simulink model "D53_LKAS_JLU_20200910_1510"  (R2018b)
settings: Solver=ode3  StartTime=0.0  StopTime=10.0  FixedStep=0.01  RelTol=1e-3  EnableMultiTasking=on
model workspace (MAT data in the model file):
  MCOS : class17 (value not decoded)
  MCOS : class17 (value not decoded)
  MCOS : class17 (value not decoded)
  MCOS : class17 (value not decoded)
  MCOS : class17 (value not decoded)
  MCOS : class17 (value not decoded)
  MCOS : class17 (value not decoded)
  MCOS : class17 (value not decoded)
  MCOS : class17 (value not decoded)
  MCOS : class17 (value not decoded)
  MCOS : class17 (value not decoded)
  MCOS : class17 (value not decoded)
  MCOS : class17 (value not decoded)
  MCOS : class17 (value not decoded)
  MCOS : class17 (value not decoded)
  MCOS : class17 (value not decoded)
  MCOS : class17 (value not decoded)
  MCOS : class17 (value not decoded)
  MCOS : class17 (value not decoded)
  MCOS : class17 (value not decoded)
  MCOS : class17 (value not decoded)
  MCOS : class17 (value not decoded)
  MCOS : class17 (value not decoded)
  MCOS : class17 (value not decoded)
  MCOS : class17 (value not decoded)
  MCOS : class17 (value not decoded)
  MCOS : class17 (value not decoded)
  MCOS : class17 (value not decoded)
  MCOS : class17 (value not decoded)
  MCOS : class17 (value not decoded)
  MCOS : class17 (value not decoded)
  MCOS : class17 (value not decoded)
  MCOS : class17 (value not decoded)
  MCOS : class17 (value not decoded)
  MCOS : class17 (value not decoded)
  MCOS : class17 (value not decoded)
  MCOS : class17 (value not decoded)
  MCOS : class17 (value not decoded)
  MCOS : class17 (value not decoded)
  MCOS : class17 (value not decoded)
  MCOS : class17 (value not decoded)
  MCOS : class17 (value not decoded)
  MCOS : class17 (value not decoded)
  MCOS : class17 (value not decoded)
  MCOS : class17 (value not decoded)
  MCOS : class17 (value not decoded)
  MCOS : class17 (value not decoded)
  MCOS : class17 (value not decoded)
  MCOS : class17 (value not decoded)
  MCOS : class17 (value not decoded)
  MCOS : class17 (value not decoded)
  MCOS : class17 (value not decoded)
  MCOS : class17 (value not decoded)
  MCOS : class17 (value not decoded)
  MCOS : class17 (value not decoded)
  MCOS : class17 (value not decoded)
  MCOS : class17 (value not decoded)
  MCOS : class17 (value not decoded)
  MCOS : class17 (value not decoded)
  MCOS : class17 (value not decoded)
  MCOS : class17 (value not decoded)
  MCOS : class17 (value not decoded)
  MCOS : class17 (value not decoded)
  MCOS : class17 (value not decoded)
  MCOS : class17 (value not decoded)
  MCOS : class17 (value not decoded)
  MCOS : class17 (value not decoded)
  MCOS : class17 (value not decoded)
  MCOS : class17 (value not decoded)
  MCOS : class17 (value not decoded)
  MCOS : class17 (value not decoded)
  MCOS : class17 (value not decoded)
  MCOS : class17 (value not decoded)
  MCOS : class17 (value not decoded)
  MCOS : class17 (value not decoded)
  MCOS : class17 (value not decoded)
  MCOS : class17 (value not decoded)
  MCOS : class17 (value not decoded)
  MCOS : class17 (value not decoded)
  MCOS : class17 (value not decoded)
  MCOS : class17 (value not decoded)
  MCOS : class17 (value not decoded)
  MCOS : class17 (value not decoded)
  MCOS : class17 (value not decoded)
  MCOS : class17 (value not decoded)
  MCOS : class17 (value not decoded)
  MCOS : class17 (value not decoded)
  MCOS : class17 (value not decoded)
  MCOS : class17 (value not decoded)
undefined symbols (not defined in the file): LKA_CarWidth, LKA_SampleTime, LKA_StrRatio_C, LKA_Veh2CamL_C, LKA_Veh2CamW_C, LKA_WhlBaseL_C, LL_CompSWA_C, LL_CrvtPrvwT_C, LL_DesDvt_C, LL_DvtComp_C, LL_DvtPrvwT_C, LL_DvtSpdDet_vDvtSpdMin_C, LL_HdAgExT_C, LL_HdAgPrvwT_C, LL_LAccMax_C, LL_LAccRMax_C, LL_LDW_EarliestWarnLine_C, LL_LDW_LatestWarnLine_C, LL_LDWS_SUPPRESS_HEADING, LL_LFClb_TFC_DiffCtlBalance, LL_LFClb_TFC_DiffCtrlMaxSWA, LL_LFClb_TFC_DiffCtrlRatio, LL_LFClb_TFC_facmGainLutGain1_C, LL_LFClb_TFC_facmGainLutGain2_C, LL_LFClb_TFC_facmIntegRatio, LL_LFClb_TFC_facmKlat_C, LL_LFClb_TFC_FfCtlRatio_C, LL_LFClb_TFC_phiIntegCtlMaxSWA_C, LL_LFClb_TFC_tiKlatPrvwT_C, LL_LFClb_TFC_vGainLutVehSpdLwr_C, LL_LFClb_TFC_vGainLutVehSpdUpr_C, LL_LKA_EarliestWarnLine_C, LL_LKA_LatestWarnLine_C, LL_LKAExPrcs_ExitC0Dvt, LL_LKAExPrcs_ExitC0Swt, LL_LKAExPrcs_tiExitTime1, LL_LKAExPrcs_tiExitTime2, LL_LKAExPrcs_tiExitTime3, LL_LKAS_OUT_OF_CONTROL_LAT_VEL, LL_LKAS_OUT_OF_CONTROL_TTLC, LL_LKASWASyn_M0, LL_LKASWASyn_M1, LL_LKASWASyn_M2, LL_LKASWASyn_M3K, LL_LKASWASyn_SWAaddMax, LL_LKASWASyn_T2, LL_LKASWASyn_tiTrqSwaRtTime, LL_LKASWASyn_tiTrqSwaTime, LL_LKASWASyn_TrqMax, LL_LKASWASyn_TrqSwaAddSwt, LL_LKASWASyn_TrqSwaRateDiff, LL_LSpdCompT_C, LL_lStpLngth_C, LL_MAX_DELAY_EPSSTAR_TIME, LL_MAX_DRIVER_TORQUE_DISABLE, LL_MAX_DRIVER_TORQUE_ENABLE, LL_MAX_LANE_WIDTH_DISABLE, LL_MAX_LANE_WIDTH_ENABLE, LL_MAX_LAT_ACC_DISABLE, LL_MAX_LAT_ACC_ENABLE ... (+30)
libraries: simulink x134, canmsglib x52, dspstat3 x3, simulink_extras x1
(part 9 of 18)

== system D53_LKAS_JLU_20200910_1510/LL/LLOn/LKA Input Processing (LKAInP)/Predicted Heading Angle Calculation (PrHdAg) ==
  PrHdAg_bsTTLCInfo : Inport
  PrdcHdAg_stLKAActvFlg : Inport  Port=2
  PrHdAg_bsInInfoSyn : Inport  Port=3
  PrHdAg_bsLKAClb : Inport  Port=4
  Add : Sum  OutDataTypeStr=single
  Add1 : Sum  OutDataTypeStr=single
  Bus Creator : BusCreator  Inputs=10
  Bus Selector : BusSelector  OutputSignals=bsLaneInfo.bsL0Info,bsVehMovInfo.ESC_VehSpd,bsLaneInfo.bsR0Info,bsSWAInfo.SW_Angle
  Bus Selector1 : BusSelector  OutputSignals=LL_HdAgPrvwT_C
  Bus Selector2 : BusSelector  OutputSignals=LFTTTLC,RGTTTLC
  Heading Angle (HdAg) : Subsystem
  Lane Information Selection (LaneInfoSel) : Subsystem
  Lane Information Selection (LaneInfoSel)1 : Subsystem
  Min : MinMax  Inputs=2
  Perdicted Heading Angle Compensation (PrdcHdAgComp) : Subsystem
  Perdicted Heading Angle from Right Lane Line (PrdcHdAgRgt) : Subsystem
  Perdicted Heading Angle from Right Lane Line (PrdcHdAgRgt)1 : Subsystem
  Predicted Heading Angle from Left Lane Line (PrdcHdAgtLft) : Subsystem
  Predicted Heading Angle from Left Lane Line (PrdcHdAgtLft)1 : Subsystem
  Saturation : Saturate  UpperLimit=2  LowerLimit=0.5
  Z Calculation (ZCalc) : Subsystem
  Z Calculation (ZCalc)1 : Subsystem
  PrHdAg_bsPrHdAgInfo : Outport
  wires:
  Perdicted Heading Angle from Right Lane Line (PrdcHdAgRgt)1/1(PrdcHdAgRgt_phiPrdcHdAgRgt) -> Bus Creator/10  "phiPrvwHdAgRgt"
  Predicted Heading Angle from Left Lane Line (PrdcHdAgtLft)1/1(PrdcHdAgtLft_phiPrdcHdAgLft) -> Bus Creator/9  "phiPrvwHdAgLft"
  Z Calculation (ZCalc)1/1(ZCalc_lPrvwDstZ) -> Predicted Heading Angle from Left Lane Line (PrdcHdAgtLft)1/2(PrdcHdAgtLft_lPrvwDstZ), Perdicted Heading Angle from Right Lane Line (PrdcHdAgRgt)1/1(PrdcHdAgRgt_lPrvwDstZ)
  Bus Selector1/1 -> Z Calculation (ZCalc)1/2(ZCalc_tiHdAgPrvwT_C)  "<LL_HdAgPrvwT_C>"
  PrHdAg_bsLKAClb/1 -> Bus Selector1/1
  Heading Angle (HdAg)/3(HdAg_phiHdAgRgt) -> Bus Creator/8  "phiHdAgRgt"
  Heading Angle (HdAg)/2(HdAg_phiHdAgLft) -> Bus Creator/7  "phiHdAgLft"
  Heading Angle (HdAg)/1(HdAg_phiHdAg) -> Bus Creator/6  "phiHdAg"
  Saturation/1 -> Perdicted Heading Angle Compensation (PrdcHdAgComp)/3(PrdcHdAgComp_tiHdAgPrvwT_C), Z Calculation (ZCalc)/2(ZCalc_tiHdAgPrvwT_C)
  Bus Selector2/2 -> Min/2  "<RGTTTLC>"
  Bus Selector2/1 -> Min/1  "<LFTTTLC>"
  PrHdAg_bsTTLCInfo/1 -> Bus Selector2/1
  Lane Information Selection (LaneInfoSel)1/1(LaneInfoSel_facmActvLane) -> Bus Creator/2  "phiPrvwTTLCHdAg"
  Bus Selector/1 -> Predicted Heading Angle from Left Lane Line (PrdcHdAgtLft)/1(PrdcHdAgtLft_bsL0Info), Predicted Heading Angle from Left Lane Line (PrdcHdAgtLft)1/1(PrdcHdAgtLft_bsL0Info)  "<bsL0Info>"
  Z Calculation (ZCalc)/1(ZCalc_lPrvwDstZ) -> Predicted Heading Angle from Left Lane Line (PrdcHdAgtLft)/2(PrdcHdAgtLft_lPrvwDstZ), Perdicted Heading Angle from Right Lane Line (PrdcHdAgRgt)/1(PrdcHdAgRgt_lPrvwDstZ)
  Lane Information Selection (LaneInfoSel)/1(LaneInfoSel_facmActvLane) -> Bus Creator/1  "phiPrdcTTLCHdAg"
  PrdcHdAg_stLKAActvFlg/1 -> Lane Information Selection (LaneInfoSel)/1(LaneInfoSel_stLKAActvFlg), Lane Information Selection (LaneInfoSel)1/1(LaneInfoSel_stLKAActvFlg)
  Add1/1 -> Lane Information Selection (LaneInfoSel)/3(LaneInfoSel_facmRgtLane)  "phiPrdcHdAgRgt"
  Add/1 -> Lane Information Selection (LaneInfoSel)/2(LaneInfoSel_facmLftLane)  "phiPrdcHdAgLft"
  Perdicted Heading Angle Compensation (PrdcHdAgComp)/1(PrdcHdAgComp_phiPrdcHdAgComp) -> Add1/2, Bus Creator/5, Add/2  "phiPrdcHdAgComp"
  Predicted Heading Angle from Left Lane Line (PrdcHdAgtLft)/1(PrdcHdAgtLft_phiPrdcHdAgLft) -> Add/1, Bus Creator/3, Lane Information Selection (LaneInfoSel)1/2(LaneInfoSel_facmLftLane)  "phiPrvwTTLCHdAgLft"
  Perdicted Heading Angle from Right Lane Line (PrdcHdAgRgt)/1(PrdcHdAgRgt_phiPrdcHdAgRgt) -> Add1/1, Lane Information Selection (LaneInfoSel)1/3(LaneInfoSel_facmRgtLane), Bus Creator/4  "phiPrvwTTLCHdAgRgt"
  Bus Creator/1 -> PrHdAg_bsPrHdAgInfo/1
  PrHdAg_bsInInfoSyn/1 -> Bus Selector/1, Heading Angle (HdAg)/1(HdAg_bsLaneInfo)
  Bus Selector/2 -> Z Calculation (ZCalc)/1(ZCalc_vVehSpd), Perdicted Heading Angle Compensation (PrdcHdAgComp)/1(PrdcHdAgComp_vVehSpd), Z Calculation (ZCalc)1/1(ZCalc_vVehSpd)  "<ESC_VehSpd>"
  Bus Selector/3 -> Perdicted Heading Angle from Right Lane Line (PrdcHdAgRgt)/2(PrdcHdAgRgt_bsR0Info), Perdicted Heading Angle from Right Lane Line (PrdcHdAgRgt)1/2(PrdcHdAgRgt_bsR0Info)  "<bsR0Info>"
  Bus Selector/4 -> Perdicted Heading Angle Compensation (PrdcHdAgComp)/2(PrdcHdAgComp_phiSWA)  "<SW_Angle>"
  Min/1 -> Saturation/1

== system D53_LKAS_JLU_20200910_1510/LL/LLOn/LKA Input Processing (LKAInP)/Previewed Curvature (PrCrvt) ==
  PrvwCrvt_stLKAActvFlg : Inport
  PrvwCrvt_bsInInfoSyn : Inport  Port=2
  PrvwCrvt_tiCrvtPrvwT_C : Inport  Port=3
  Bus Creator : BusCreator  Inputs=3
  Bus Selector : BusSelector  OutputSignals=LL_CrvtPrvwT_C
  Bus Selector2 : BusSelector  OutputSignals=bsLaneInfo.bsL0Info,bsVehMovInfo.ESC_VehSpd,bsLaneInfo.bsR0Info
  Curvature Ahead of Left Lane Line (CrvtAhdLft) : Subsystem
  Curvature Ahead of Left Lane Line (CrvtAhdLft)1 : Subsystem
  Lane Information Selection (LaneInfoSel) : Subsystem
  Z Calculation (ZCalc) : Subsystem
  PrvwCrvt_bsPrvwCrvtInfo : Outport
  wires:
  Bus Creator/1 -> PrvwCrvt_bsPrvwCrvtInfo/1
  Lane Information Selection (LaneInfoSel)/1(LaneInfoSel_facmActvLane) -> Bus Creator/1  "crPrvwCrvt"
  Curvature Ahead of Left Lane Line (CrvtAhdLft)1/1(CrvtAhdRgt_crCrvtAhdRgt) -> Bus Creator/3, Lane Information Selection (LaneInfoSel)/3(LaneInfoSel_facmRgtLane)  "crPrvwCrvtRgt"
  Curvature Ahead of Left Lane Line (CrvtAhdLft)/1(CrvtAhdLft_crCrvtAhdLft) -> Lane Information Selection (LaneInfoSel)/2(LaneInfoSel_facmLftLane), Bus Creator/2  "crPrvwCrvtLft"
  PrvwCrvt_stLKAActvFlg/1 -> Lane Information Selection (LaneInfoSel)/1(LaneInfoSel_stLKAActvFlg)
  Bus Selector/1 -> Z Calculation (ZCalc)/2(ZCalc_tiCrvtPrvwT_C)  "<LL_CrvtPrvwT_C>"
  PrvwCrvt_tiCrvtPrvwT_C/1 -> Bus Selector/1
  Bus Selector2/2 -> Z Calculation (ZCalc)/1(ZCalc_vVehSpd)  "<ESC_VehSpd>"
  Bus Selector2/3 -> Curvature Ahead of Left Lane Line (CrvtAhdLft)1/2(CrvtAhdRgt_bsR0Info)  "<bsR0Info>"
  Bus Selector2/1 -> Curvature Ahead of Left Lane Line (CrvtAhdLft)/1(CrvtAhdLft_bsL0Info)  "<bsL0Info>"
  Z Calculation (ZCalc)/1(ZCalc_lPrvwDstZ) -> Curvature Ahead of Left Lane Line (CrvtAhdLft)/2(CrvtAhdLft_lPrvwDstZ), Curvature Ahead of Left Lane Line (CrvtAhdLft)1/1(CrvtAhdRgt_lPrvwDstZ)
  PrvwCrvt_bsInInfoSyn/1 -> Bus Selector2/1

== system D53_LKAS_JLU_20200910_1510/LL/LLOn/LKA Input Processing (LKAInP)/Steering Wheel Position Calculation (SWAPosCal) ==
  SWAPosCal_bsInInfoSyn : Inport
  Bus Selector : BusSelector  OutputSignals=bsLaneInfo.bsL0Info,bsLaneInfo.bsR0Info,bsVehMovInfo.ESC_VehSpd,bsSWAInfo.SW_Angle
  Bus Selector2 : BusSelector  OutputSignals=LKA_SampleTime
  Subsystem : Subsystem
  Subsystem1 : Subsystem
  SWAPosCal : Outport
  wires:
  Bus Selector2/1 -> Subsystem/2(<LKA_SampleTime>)  "<LKA_SampleTime>"
  [LLClb_bsConstantClb] -> Bus Selector2/1
  Subsystem/1(SWAPos) -> SWAPosCal/1
  Bus Selector/4 -> Subsystem1/4(SWA), Subsystem/1(SWAIn)  "<SW_Angle>"
  Bus Selector/3 -> Subsystem1/3(VehSpd)  "<ESC_VehSpd>"
  Subsystem1/1(Flg) -> Subsystem/Enable  "SWAPosEna"
  Bus Selector/2 -> Subsystem1/2(R0)  "<bsR0Info>"
  Bus Selector/1 -> Subsystem1/1(L0)  "<bsL0Info>"
  SWAPosCal_bsInInfoSyn/1 -> Bus Selector/1

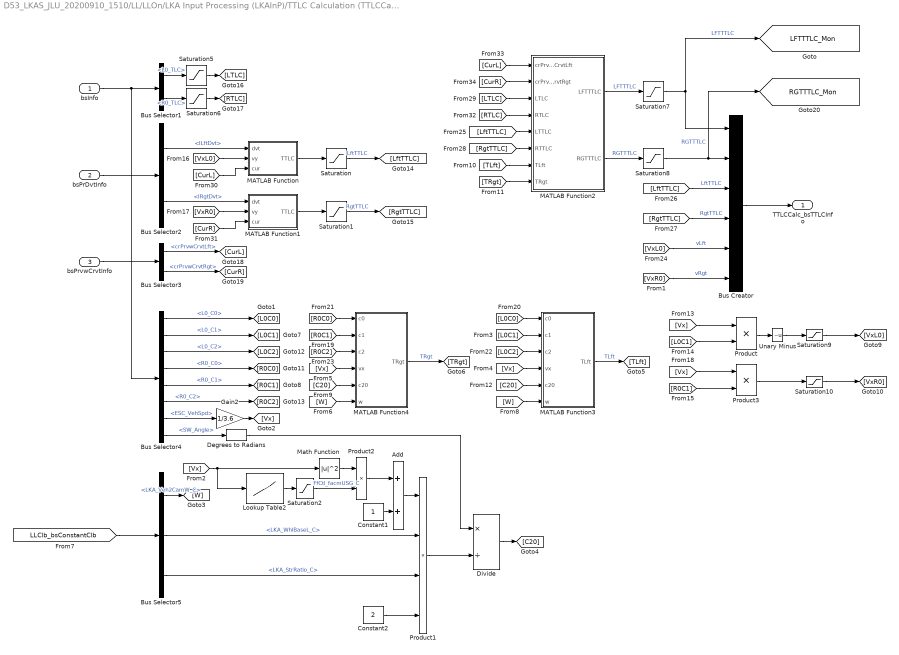
== system D53_LKAS_JLU_20200910_1510/LL/LLOn/LKA Input Processing (LKAInP)/TTLC Calculation (TTLCCalc) ==
  bsInfo : Inport
  bsPrDvtInfo : Inport  Port=2
  bsPrvwCrvtInfo : Inport  Port=3
  Add : Sum  OutDataTypeStr=single
  Bus Creator : BusCreator  Inputs=6
  Bus Selector1 : BusSelector  OutputSignals=bsLaneInfo.bsL0Info.L0_TLC,bsLaneInfo.bsR0Info.R0_TLC
  Bus Selector2 : BusSelector  OutputSignals=ILftDvt,IRgtDvt
  Bus Selector3 : BusSelector  OutputSignals=crPrvwCrvtLft,crPrvwCrvtRgt
  Bus Selector4 : BusSelector  OutputSignals=bsLaneInfo.bsL0Info.L0_C0,bsLaneInfo.bsL0Info.L0_C1,bsLaneInfo.bsL0Info.L0_C2,bsLaneInfo.bsR0Info.R0_C0,bsLaneInfo.bsR0Info.R0_C1,bsLaneInfo.bsR0Info.R0_C2,bsVehMovInfo.ESC_VehSpd,bsSWAInfo.SW_Angle
  Bus Selector5 : BusSelector  OutputSignals=LKA_Veh2CamW_C,LKA_WhlBaseL_C,LKA_StrRatio_C
  Constant1 : Constant  OutDataTypeStr=single
  Constant2 : Constant  Value=2  OutDataTypeStr=single
  Degrees to Radians : simulink_extras/Transformations/Degrees to Radians
  Divide : Product  Inputs=*/
  Gain2 : Gain  Gain=1/3.6
  Lookup Table2 : Lookup_n-D  NumberOfTableDimensions=1  BreakpointsForDimension1=[11.7,18.83,26.98,31.98,51.04,79,86.08,90.59]  BeginIndexSearchUsingPreviousIndexResult=on  Table=[0.012141,0.005179,0.00298,0.002547,0.001715,0.001283,0.001021,0.000982]  DiagnosticForOutOfRangeInput=Warning  RemoveProtectionInput=on  InternalRulePriority=Speed  OutDataTypeStr=single  RndMeth=Simplest  InputSameDT=on
  MATLAB Function : MATLAB Function  TreatAsAtomicUnit=on
  MATLAB Function1 : MATLAB Function  TreatAsAtomicUnit=on
  MATLAB Function2 : MATLAB Function  TreatAsAtomicUnit=on
  MATLAB Function3 : MATLAB Function  TreatAsAtomicUnit=on
  MATLAB Function4 : MATLAB Function  TreatAsAtomicUnit=on
  Math Function : Math  Operator=magnitude^2  OutDataTypeStr=single  SaturateOnIntegerOverflow=on
  Product : Product
  Product1 : Product  Inputs=4  OutDataTypeStr=single
  Product2 : Product  OutDataTypeStr=single
  Product3 : Product
  Saturation : Saturate  UpperLimit=2  LowerLimit=0.6  OutDataTypeStr=single
  Saturation1 : Saturate  UpperLimit=2  LowerLimit=0.6  OutDataTypeStr=single
  Saturation10 : Saturate  UpperLimit=1  LowerLimit=-1
  Saturation2 : Saturate  UpperLimit=0.01  LowerLimit=0
  Saturation5 : Saturate  UpperLimit=2  LowerLimit=0.6
  Saturation6 : Saturate  UpperLimit=2  LowerLimit=0.6
  Saturation7 : Saturate  UpperLimit=2  LowerLimit=0.8
  Saturation8 : Saturate  UpperLimit=2  LowerLimit=0.8
  Saturation9 : Saturate  UpperLimit=1  LowerLimit=-1
  Unary Minus : UnaryMinus
  TTLCCalc_bsTTLCInfo : Outport
  tag scope: LFTTTLC_Mon=global, RGTTTLC_Mon=global
  wires:
  Constant2/1 -> Product1/4
  [CurR] -> MATLAB Function2/2(crPrvwCrvtRgt)
  Saturation8/1 -> Bus Creator/2, [RGTTTLC_Mon]  "RGTTTLC"
  MATLAB Function2/2(RGTTTLC) -> Saturation8/1  "RGTTTLC"
  [LTLC] -> MATLAB Function2/3(LTLC)
  [RgtTTLC] -> MATLAB Function2/6(RTTLC)
  [RgtTTLC] -> Bus Creator/4  "RgtTTLC"
  [RTLC] -> MATLAB Function2/4(RTLC)
  MATLAB Function2/1(LFTTTLC) -> Saturation7/1  "LFTTTLC"
  [CurL] -> MATLAB Function2/1(crPrvwCrvtLft)
  Saturation7/1 -> Bus Creator/1, [LFTTTLC_Mon]  "LFTTTLC"
  [LftTTLC] -> Bus Creator/3  "LftTTLC"
  [TRgt] -> MATLAB Function2/8(TRgt)
  [LftTTLC] -> MATLAB Function2/5(LTTLC)
  [TLft] -> MATLAB Function2/7(TLft)
  Bus Creator/1 -> TTLCCalc_bsTTLCInfo/1
  [VxL0] -> Bus Creator/5  "vLft"
  [VxR0] -> Bus Creator/6  "vRgt"
  Saturation10/1 -> [VxR0]
  Unary Minus/1 -> Saturation9/1
  [R0C1] -> Product3/2
  Product/1 -> Unary Minus/1
  Saturation9/1 -> [VxL0]
  [Vx] -> Product/1
  [L0C1] -> Product/2
  [Vx] -> Product3/1
  Product3/1 -> Saturation10/1
  [L0C0] -> MATLAB Function3/1(c0)
  [L0C2] -> MATLAB Function3/3(c2)
  [Vx] -> MATLAB Function4/4(vx)
  [R0C1] -> MATLAB Function4/2(c1)
  [W] -> MATLAB Function3/6(w)
  [L0C1] -> MATLAB Function3/2(c1)
  MATLAB Function3/1(TLft) -> [TLft]  "TLft"
  [R0C0] -> MATLAB Function4/1(c0)
  [W] -> MATLAB Function4/6(w)
  [C20] -> MATLAB Function4/5(c20)
  [Vx] -> MATLAB Function3/4(vx)
  [R0C2] -> MATLAB Function4/3(c2)
  MATLAB Function4/1(TRgt) -> [TRgt]  "TRgt"
  [C20] -> MATLAB Function3/5(c20)
  Bus Selector4/3 -> [L0C2]  "<L0_C2>"
  Bus Selector4/1 -> [L0C0]  "<L0_C0>"
  Bus Selector4/2 -> [L0C1]  "<L0_C1>"
  Bus Selector4/6 -> [R0C2]  "<R0_C2>"
  Bus Selector4/4 -> [R0C0]  "<R0_C0>"
  Bus Selector4/5 -> [R0C1]  "<R0_C1>"
  Bus Selector3/2 -> [CurR]  "<crPrvwCrvtRgt>"
  Bus Selector3/1 -> [CurL]  "<crPrvwCrvtLft>"
  [CurL] -> MATLAB Function/3(cur)
  [CurR] -> MATLAB Function1/3(cur)
  Bus Selector2/1 -> MATLAB Function/1(dvt)  "<ILftDvt>"
  Saturation1/1 -> [RgtTTLC]  "RgtTTLC"
  Saturation/1 -> [LftTTLC]  "LftTTLC"
  MATLAB Function/1(TTLC) -> Saturation/1
  MATLAB Function1/1(TTLC) -> Saturation1/1
  [VxR0] -> MATLAB Function1/2(vy)
  [VxL0] -> MATLAB Function/2(vy)
  Bus Selector2/2 -> MATLAB Function1/1(dvt)  "<IRgtDvt>"
  Bus Selector1/2 -> Saturation6/1  "<R0_TLC>"
  Bus Selector1/1 -> Saturation5/1  "<L0_TLC>"
  Saturation5/1 -> [LTLC]
  Saturation6/1 -> [RTLC]
  bsPrvwCrvtInfo/1 -> Bus Selector3/1
  bsPrDvtInfo/1 -> Bus Selector2/1
  bsInfo/1 -> Bus Selector4/1, Bus Selector1/1
  [LLClb_bsConstantClb] -> Bus Selector5/1
  Product2/1 -> Add/1
  Math Function/1 -> Product2/1
  Lookup Table2/1 -> Saturation2/1
  Constant1/1 -> Add/2
  Saturation2/1 -> Product2/2  "FfCtl_facmUSG_C"
  Bus Selector4/7 -> Gain2/1  "<ESC_VehSpd>"
  Add/1 -> Product1/1
  Bus Selector5/2 -> Product1/2  "<LKA_WhlBaseL_C>"
  Bus Selector5/3 -> Product1/3  "<LKA_StrRatio_C>"
  Product1/1 -> Divide/2
  Bus Selector4/8 -> Degrees to Radians/1  "<SW_Angle>"
  Degrees to Radians/1 -> Divide/1
  Gain2/1 -> [Vx]
  [Vx] -> Lookup Table2/1, Math Function/1
  Bus Selector5/1 -> [W]  "<LKA_Veh2CamW_C>"
  Divide/1 -> [C20]

== system D53_LKAS_JLU_20200910_1510/LL/LLOn/LKA Input Processing (LKAInP)/Under The Limit (UndrLim) ==
  UndrLim_bsInInfoSyn : Inport
  UndrLim_bsUndrLimClb : Inport  Port=2
  Bus Selector : BusSelector  OutputSignals=LL_LAccMax_C,LL_LAccRMax_C
  Bus Selector1 : BusSelector  OutputSignals=bsVehMovInfo.ESC_VehSpd
  Bus Selector2 : BusSelector  OutputSignals=LKA_StrRatio_C,LKA_WhlBaseL_C
  Saturation : Saturate  UpperLimit=150  LowerLimit=0.001
  Steering Wheel Angel Max (SWAMax) : Subsystem
  Steering Wheel Angel Rate Max (SWARMax) : Subsystem
  UndrLim_phiSWAMax : Outport
  UndrLim_dphiSWARMax : Outport  Port=2
  wires:
  [LLClb_bsConstantClb] -> Bus Selector2/1
  Bus Selector2/2 -> Steering Wheel Angel Rate Max (SWARMax)/4(LKA_WhlBaseL_C), Steering Wheel Angel Max (SWAMax)/4(LKA_WhlBaseL_C)  "<LKA_WhlBaseL_C>"
  Bus Selector2/1 -> Steering Wheel Angel Rate Max (SWARMax)/3(LKA_StrRatio_C), Steering Wheel Angel Max (SWAMax)/3(LKA_StrRatio_C)  "<LKA_StrRatio_C>"
  Bus Selector1/1 -> Saturation/1  "<ESC_VehSpd>"
  UndrLim_bsInInfoSyn/1 -> Bus Selector1/1
  Bus Selector/2 -> Steering Wheel Angel Rate Max (SWARMax)/2(SWARateMax_aLAccR_C)  "<LL_LAccRMax_C>"
  Bus Selector/1 -> Steering Wheel Angel Max (SWAMax)/2(SWAMax_aLAcc_C)  "<LL_LAccMax_C>"
  UndrLim_bsUndrLimClb/1 -> Bus Selector/1
  Steering Wheel Angel Max (SWAMax)/1(SWAMax_phiSWAMax) -> UndrLim_phiSWAMax/1
  Steering Wheel Angel Rate Max (SWARMax)/1(SWARMax_dphiSWARMax) -> UndrLim_dphiSWARMax/1
  Saturation/1 -> Steering Wheel Angel Max (SWAMax)/1(SWAMax_vVehSpd), Steering Wheel Angel Rate Max (SWARMax)/1(SWARateMax_vVehSpd)

== system D53_LKAS_JLU_20200910_1510/LL/LLOn/LL State Determination (LLStateDet)/LL State Machine Conditions (LLSMCon) ==
  LLSMCon_stDACModeIn : Inport
  LLSMCon_bsInInfoSyn : Inport  Port=2
  LLSMCon_bsLKAInPInfo : Inport  Port=3
  LLSMCon_bsLLSMConClb : Inport  Port=4
  LLSMCon_bsLLState : Inport  Port=5
  LLSMCon_stExitFlg : Inport  Port=6
  LLSMCon_bsSignalFault : Inport  Port=7
  Activation Condition (ActvC) : Subsystem  Description=|
      | Block Name: Activation Condition
      | Ab.: ActvC
      | No.: 1.1.1.4.0.
      | Rev: 0.0.1
      | Update Date: 19-3-26
  Deactivation Condition (DeactvC) : Subsystem  Description=|
      | Block Name: Deactivation Condition
      | Ab.: DeactvC
      | No.: 1.1.1.5.0.0
      | Rev: 0.0.1
      | Update Date: 19-3-26
  Disable Condition (DisblC) : Subsystem  Description=|
      | Block Name: Disable Condition
      | Ab.: DisblC
      | No.: 1.1.1.3.0.0
      | Rev: 0.0.1
      | Update Date: 19-3-26
  Enable Condition (EnaC) : Subsystem  Description=|
      | Block Name: Enable Condition
      | Ab.: EnaC
      | No.: 1.1.1.2.0.0
      | Rev: 0.0.1
      | Update Date: 19-3-26
      settings: PermitHierarchicalResolution=None  MinAlgLoopOccurrences=on
  Fault Condition (FaultC) : Subsystem  Description=|
      | Block Name: Fault Condition
      | Ab.: FaultC
      | No.: 1.1.1.6.0.0
      | Rev: 0.0.1
      | Update Date: 19-3-26
  LLSMCon_stDACMode : Outport
  LLSMCon_stLDWEnaCSyn : Outport  Port=2
  LLSMCon_stLDWDisblCSyn : Outport  Port=3
  LLSMCon_stLDWActvCSyn : Outport  Port=4
  LLSMCon_stLDWDeactvCSyn : Outport  Port=5
  LLSMCon_stLDWFaultCSyn : Outport  Port=6
  LLSMCon_stLKAEnaCSyn : Outport  Port=7
  LLSMCon_stLKADisblCSyn : Outport  Port=8
  LLSMCon_stLKAActvCSyn : Outport  Port=9
  LLSMCon_stLKADeactvCSyn : Outport  Port=10
  LLSMCon_stLKAFaultCSyn : Outport  Port=11
  wires:
  LLSMCon_bsLKAInPInfo/1 -> Enable Condition (EnaC)/3(EnaC_bsLKAInPInfo), Disable Condition (DisblC)/3(LKAInPInfo), Activation Condition (ActvC)/3(LKAInPInfo), Deactivation Condition (DeactvC)/3(LKAInPInfo)
  LLSMCon_bsSignalFault/1 -> Fault Condition (FaultC)/2(FaultC_SignalFault)
  Activation Condition (ActvC)/2(ActvC_stLKAActvCSyn) -> LLSMCon_stLKAActvCSyn/1
  LLSMCon_bsLLSMConClb/1 -> Enable Condition (EnaC)/4(EnaC_bsLLSMConClb), Disable Condition (DisblC)/4(LLSMConClb), Activation Condition (ActvC)/4(LLSMConClb), Deactivation Condition (DeactvC)/4(LLSMConClb)
  LLSMCon_stExitFlg/1 -> Deactivation Condition (DeactvC)/6(ExitFlg)
  Deactivation Condition (DeactvC)/1(DeactvC_stLDWDeactvCSyn) -> LLSMCon_stLDWDeactvCSyn/1
  Fault Condition (FaultC)/2(FaultC_stLKAFaultCSyn) -> LLSMCon_stLKAFaultCSyn/1
  Deactivation Condition (DeactvC)/2(DeactvC_stLKADeactvCSyn) -> LLSMCon_stLKADeactvCSyn/1
  Fault Condition (FaultC)/1(FaultC_stLDWFaultCSyn) -> LLSMCon_stLDWFaultCSyn/1
  LLSMCon_stDACModeIn/1 -> Enable Condition (EnaC)/1(EnaC_stDACMode), Disable Condition (DisblC)/1(DACMode), Activation Condition (ActvC)/1(DACMode), Deactivation Condition (DeactvC)/1(DACMode), LLSMCon_stDACMode/1
  Activation Condition (ActvC)/1(ActvC_stLDWActvCSyn) -> LLSMCon_stLDWActvCSyn/1
  LLSMCon_bsInInfoSyn/1 -> Disable Condition (DisblC)/2(InInfoSyn), Activation Condition (ActvC)/2(InInfoSyn), Deactivation Condition (DeactvC)/2(InInfoSyn), Fault Condition (FaultC)/1(FaultC_bsInInfoSyn), Enable Condition (EnaC)/2(EnaC_bsInInfoSyn)
  LLSMCon_bsLLState/1 -> Disable Condition (DisblC)/5(LLState), Deactivation Condition (DeactvC)/5(LLState)
  Enable Condition (EnaC)/1(EnaC_stLDWEnaCSyn) -> LLSMCon_stLDWEnaCSyn/1
  Disable Condition (DisblC)/2(DisblC_stLKADisblCSyn) -> LLSMCon_stLKADisblCSyn/1
  Disable Condition (DisblC)/1(DisblC_stLDWDisblCSyn) -> LLSMCon_stLDWDisblCSyn/1
  Enable Condition (EnaC)/2(EnaC_stLKAEnaCSyn) -> LLSMCon_stLKAEnaCSyn/1

== system D53_LKAS_JLU_20200910_1510/LL/LL Inputs Mapping/bsLaneInfo/LaneSelect/Subsystem ==
  R0_Q_In : Inport
  Constant1 : Constant  Value=3  OutDataTypeStr=uint8
  Switch1 : Switch  Threshold=2
  R0_Q : Outport
  wires:
  Constant1/1 -> Switch1/1
  R0_Q_In/1 -> Switch1/2, Switch1/3
  Switch1/1 -> R0_Q/1  "R0_Q"

== system D53_LKAS_JLU_20200910_1510/LL/LL Inputs Mapping/bsLaneInfo/LaneSelect/Subsystem1 ==
  R0_Q_In : Inport
  Constant1 : Constant  Value=3  OutDataTypeStr=uint8
  Switch1 : Switch  Threshold=2
  R0_Q : Outport
  wires:
  Switch1/1 -> R0_Q/1  "R0_Q"
  R0_Q_In/1 -> Switch1/3, Switch1/2
  Constant1/1 -> Switch1/1

== system D53_LKAS_JLU_20200910_1510/LL/LL Inputs Mapping/bsLaneInfo/LaneSelect/Subsystem2 ==
  L0_Q_In : Inport
  Constant : Constant  Value=3  OutDataTypeStr=uint8
  Switch : Switch  Threshold=2
  L0_Q : Outport
  wires:
  Switch/1 -> L0_Q/1  "L0_Q"
  Constant/1 -> Switch/1
  L0_Q_In/1 -> Switch/2, Switch/3

== system D53_LKAS_JLU_20200910_1510/LL/LL Inputs Mapping/bsLaneInfo/LaneSelect/Subsystem4 ==
  L0_Q_In : Inport
  Constant : Constant  Value=3  OutDataTypeStr=uint8
  Switch : Switch  Threshold=2
  L0_Q : Outport
  wires:
  L0_Q_In/1 -> Switch/3, Switch/2
  Constant/1 -> Switch/1
  Switch/1 -> L0_Q/1  "L0_Q"

== system D53_LKAS_JLU_20200910_1510/LL/LL Inputs Mapping/bsLaneInfo/LanesReconstruct /Left 1Lane Reconstruct (Lft1LaneR) ==
  stFlag : Inport
  bsL1Info : Inport  Port=2
  Bus Creator2 : BusCreator  Inputs=10
  Bus Selector1 : BusSelector  OutputSignals=L1_C0,L1_C1,L1_C2,L1_C3,L1_VR,L1_Q,L1_Type,L1_W,L1_TLC,L1_LC
  Constant : Constant  Value=0  OutDataTypeStr=uint16
  Switch3 : Switch  Criteria=u2 > Threshold
  bsL1InfoR : Outport
  wires:
  Bus Selector1/1 -> Bus Creator2/1  "<L1_C0>"
  Bus Selector1/2 -> Bus Creator2/2  "<L1_C1>"
  Bus Selector1/3 -> Bus Creator2/3  "<L1_C2>"
  Bus Selector1/4 -> Bus Creator2/4  "<L1_C3>"
  Bus Creator2/1 -> bsL1InfoR/1  "bsL1Info"
  Switch3/1 -> Bus Creator2/6  "L1_Q"
  Constant/1 -> Switch3/3
  Bus Selector1/6 -> Switch3/1  "<L1_Q>"
  stFlag/1 -> Switch3/2
  bsL1Info/1 -> Bus Selector1/1
  Bus Selector1/5 -> Bus Creator2/5  "<L1_VR>"
  Bus Selector1/7 -> Bus Creator2/7  "<L1_Type>"
  Bus Selector1/8 -> Bus Creator2/8  "<L1_W>"
  Bus Selector1/10 -> Bus Creator2/10  "<L1_LC>"
  Bus Selector1/9 -> Bus Creator2/9  "<L1_TLC>"

== system D53_LKAS_JLU_20200910_1510/LL/LL Inputs Mapping/bsLaneInfo/LanesReconstruct /Left Lane Reconstruct (LftLaneR) ==
  lRoadW : Inport
  bsR0Info : Inport  Port=2
  bsL0Info : Inport  Port=3
  Add : Sum  Inputs=+-  OutDataTypeStr=single
  Bus Creator : BusCreator  Inputs=10
  Bus Selector1 : BusSelector  OutputSignals=L0_Q
  Bus Selector3 : BusSelector  OutputSignals=R0_C0,R0_C1,R0_C2,R0_C3,R0_VR,R0_Type,R0_W,R0_TLC,R0_LC
  Cast To Single{1..4,6..7} (6 alike) : DataTypeConversion  OutDataTypeStr=single  LockScale=on
  Cast To Single5 : DataTypeConversion  OutDataTypeStr=uint8  LockScale=on
  Cast To Single8 : DataTypeConversion  OutDataTypeStr=uint8  LockScale=on
  Gain : Gain  Gain=-1  OutDataTypeStr=Inherit: Same as input
  bsL0InfoR : Outport
  wires:
  Bus Creator/1 -> bsL0InfoR/1  "bsL0Info"
  Cast To Single3/1 -> Bus Creator/4  "L0_C3"
  Cast To Single2/1 -> Bus Creator/3  "L0_C2"
  Cast To Single1/1 -> Bus Creator/2  "L0_C1"
  Gain/1 -> Bus Creator/1  "L0_C0"
  Bus Selector1/1 -> Bus Creator/6  "<L0_Q>"
  bsL0Info/1 -> Bus Selector1/1
  Bus Selector3/5 -> Cast To Single4/1  "<R0_VR>"
  Bus Selector3/4 -> Cast To Single3/1  "<R0_C3>"
  Bus Selector3/3 -> Cast To Single2/1  "<R0_C2>"
  Bus Selector3/2 -> Cast To Single1/1  "<R0_C1>"
  Add/1 -> Gain/1
  Bus Selector3/1 -> Add/2  "<R0_C0>"
  bsR0Info/1 -> Bus Selector3/1
  lRoadW/1 -> Add/1
  Bus Selector3/6 -> Cast To Single5/1  "<R0_Type>"
  Bus Selector3/7 -> Cast To Single6/1  "<R0_W>"
  Bus Selector3/9 -> Cast To Single8/1  "<R0_LC>"
  Bus Selector3/8 -> Cast To Single7/1  "<R0_TLC>"
  Cast To Single5/1 -> Bus Creator/7  "L0_Type"
  Cast To Single6/1 -> Bus Creator/8  "L0_W"
  Cast To Single4/1 -> Bus Creator/5  "L0_VR"
  Cast To Single8/1 -> Bus Creator/10  "L0_LC"
  Cast To Single7/1 -> Bus Creator/9  "L0_TLC"

== system D53_LKAS_JLU_20200910_1510/LL/LL Inputs Mapping/bsLaneInfo/LanesReconstruct /Right 1Lane Reconstruct (Rgt1LaneR) ==
  stFlag : Inport
  bsR1Info : Inport  Port=2
  Bus Creator3 : BusCreator  Inputs=10
  Bus Selector1 : BusSelector  OutputSignals=R1_C0,R1_C1,R1_C2,R1_C3,R1_VR,R1_Q,R1_Type,R1_W,R1_TLC,R1_LC
  Constant : Constant  Value=0  OutDataTypeStr=uint16
  Switch3 : Switch  Criteria=u2 > Threshold
  bsL1InfoR : Outport
  wires:
  Switch3/1 -> Bus Creator3/6  "R1_Q"
  Bus Creator3/1 -> bsL1InfoR/1  "bsR1Info"
  bsR1Info/1 -> Bus Selector1/1
  stFlag/1 -> Switch3/2
  Bus Selector1/6 -> Switch3/1  "<R1_Q>"
  Constant/1 -> Switch3/3
  Bus Selector1/4 -> Bus Creator3/4  "<R1_C3>"
  Bus Selector1/3 -> Bus Creator3/3  "<R1_C2>"
  Bus Selector1/2 -> Bus Creator3/2  "<R1_C1>"
  Bus Selector1/1 -> Bus Creator3/1  "<R1_C0>"
  Bus Selector1/5 -> Bus Creator3/5  "<R1_VR>"
  Bus Selector1/7 -> Bus Creator3/7  "<R1_Type>"
  Bus Selector1/8 -> Bus Creator3/8  "<R1_W>"
  Bus Selector1/10 -> Bus Creator3/10  "<R1_LC>"
  Bus Selector1/9 -> Bus Creator3/9  "<R1_TLC>"

== system D53_LKAS_JLU_20200910_1510/LL/LL Inputs Mapping/bsLaneInfo/LanesReconstruct /Right Lane Reconstruct (RgtLaneR) ==
  bsL0Info : Inport
  bsR0Info : Inport  Port=2
  lRoadW : Inport  Port=3
  Add : Sum  OutDataTypeStr=single
  Bus Creator1 : BusCreator  Inputs=10
  Bus Selector1 : BusSelector  OutputSignals=R0_Q
  Bus Selector3 : BusSelector  OutputSignals=L0_C0,L0_C1,L0_C2,L0_C3,L0_VR,L0_Type,L0_W,L0_TLC,L0_LC
  Cast To Single{1..4,6..7} (6 alike) : DataTypeConversion  OutDataTypeStr=single  LockScale=on
  Cast To Single5 : DataTypeConversion  OutDataTypeStr=uint8  LockScale=on
  Cast To Single8 : DataTypeConversion  OutDataTypeStr=uint8  LockScale=on
  bsR0InfoR : Outport
  wires:
  Cast To Single4/1 -> Bus Creator1/5  "R0_VR"
  Cast To Single3/1 -> Bus Creator1/4  "R0_C3"
  Cast To Single2/1 -> Bus Creator1/3  "R0_C2"
  Cast To Single1/1 -> Bus Creator1/2  "R0_C1"
  Add/1 -> Bus Creator1/1  "R0_C0"
  Bus Creator1/1 -> bsR0InfoR/1  "bsR0Info"
  Bus Selector1/1 -> Bus Creator1/6  "<R0_Q>"
  bsR0Info/1 -> Bus Selector1/1
  Bus Selector3/5 -> Cast To Single4/1  "<L0_VR>"
  Bus Selector3/4 -> Cast To Single3/1  "<L0_C3>"
  Bus Selector3/3 -> Cast To Single2/1  "<L0_C2>"
  Bus Selector3/2 -> Cast To Single1/1  "<L0_C1>"
  lRoadW/1 -> Add/1
  bsL0Info/1 -> Bus Selector3/1
  Bus Selector3/1 -> Add/2  "<L0_C0>"
  Bus Selector3/6 -> Cast To Single5/1  "<L0_Type>"
  Bus Selector3/7 -> Cast To Single6/1  "<L0_W>"
  Bus Selector3/9 -> Cast To Single8/1  "<L0_LC>"
  Bus Selector3/8 -> Cast To Single7/1  "<L0_TLC>"
  Cast To Single5/1 -> Bus Creator1/7  "R0_Type"
  Cast To Single8/1 -> Bus Creator1/10  "R0_LC"
  Cast To Single6/1 -> Bus Creator1/8  "R0_W"
  Cast To Single7/1 -> Bus Creator1/9  "R0_TLC"

== system D53_LKAS_JLU_20200910_1510/LL/LL Inputs Mapping/bsLaneInfo/LanesReconstruct /RoadSide Offset ==
  bsL0Info : Inport
  bsR0Info : Inport  Port=2
  Abs : Abs
  Add : Sum
  Add1 : Sum  Inputs=+-
  Add2 : Sum
  Average Filter (AvrgFlt) : Subsystem
      mask Display:
      | port_label('input', 1, 'In');
      | port_label('input', 2, 'PtsNum');
      | port_label('output', 1, 'Out');
      | color('blue');
      | text(0.98,0.9,'VCDC Block','horizontalAlignment','right');
      | color('black');
      | text(0.5,0.55,'Average Filter','horizontalAlignment','center');
      | text(0.5,0.4,'(AvrgFlt)','horizontalAlignment','center');
  Average Filter (AvrgFlt)1 : Subsystem
      mask Display:
      | port_label('input', 1, 'In');
      | port_label('input', 2, 'PtsNum');
      | port_label('output', 1, 'Out');
      | color('blue');
      | text(0.98,0.9,'VCDC Block','horizontalAlignment','right');
      | color('black');
      | text(0.5,0.55,'Average Filter','horizontalAlignment','center');
      | text(0.5,0.4,'(AvrgFlt)','horizontalAlignment','center');
  Bus Creator1 : BusCreator  Inputs=10
  Bus Creator2 : BusCreator  Inputs=10
  Bus Selector1 : BusSelector  OutputSignals=R0_C0,R0_C1,R0_C2,R0_C3,R0_VR,R0_Q,R0_Type,R0_W,R0_TLC,R0_LC
  Bus Selector3 : BusSelector  OutputSignals=L0_C0,L0_C1,L0_C2,L0_C3,L0_VR,L0_Q,L0_Type,L0_W,L0_TLC,L0_LC
  Compare To Constant : simulink/Logic and Bit Operations/Compare To Constant  relop===  const=2  OutDataTypeStr=boolean
  Compare To Constant1 : simulink/Logic and Bit Operations/Compare To Constant  relop===  const=2  OutDataTypeStr=boolean
  PtsNum : Constant  Value=10  OutDataTypeStr=single
  PtsNum1 : Constant  Value=10  OutDataTypeStr=single
  Road Width Calculation (RoadWCal) : Subsystem
  Saturation : Saturate  UpperLimit=0.004  LowerLimit=0
  Switch : Switch  Criteria=u2 > Threshold
  Switch1 : Switch  Criteria=u2 > Threshold
  get_roadside_offset : MATLAB Function  TreatAsAtomicUnit=on
  bsL0Infoout : Outport
  bsR0Infoout : Outport  Port=2
  lRoadW : Outport  Port=3
  wires:
  PtsNum1/1 -> Average Filter (AvrgFlt)1/2(PtsNum)
  Switch1/1 -> Average Filter (AvrgFlt)1/1(In)
  PtsNum/1 -> Average Filter (AvrgFlt)/2(PtsNum)
  Switch/1 -> Average Filter (AvrgFlt)/1(In)
  get_roadside_offset/1(offset) -> [offset]
  Saturation/1 -> get_roadside_offset/1(cur)
  Abs/1 -> Saturation/1
  Add2/1 -> Abs/1
  Road Width Calculation (RoadWCal)/1(RoadWCal_lRoadW) -> get_roadside_offset/2(lanewidth), lRoadW/1
  Bus Selector1/1 -> Add1/1, Switch1/3  "<R0_C0>"
  [offset] -> Add1/2
  Compare To Constant1/1 -> Switch1/2
  Average Filter (AvrgFlt)1/1(Out) -> Bus Creator2/1  "R0_C0"
  Bus Selector1/8 -> Bus Creator2/8  "<R0_W>"
  Add1/1 -> Switch1/1
  Bus Selector1/7 -> Compare To Constant1/1, Bus Creator2/7  "<R0_Type>"
  Bus Selector1/10 -> Bus Creator2/10  "<R0_LC>"
  Bus Selector1/6 -> Bus Creator2/6  "<R0_Q>"
  Bus Selector1/4 -> Bus Creator2/4  "<R0_C3>"
  Bus Creator2/1 -> bsR0Infoout/1  "bsR0Info"
  Bus Selector1/2 -> Bus Creator2/2  "<R0_C1>"
  Bus Selector1/5 -> Bus Creator2/5  "<R0_VR>"
  bsR0Info/1 -> Bus Selector1/1, Road Width Calculation (RoadWCal)/2(RoadWCal_R0Info)
  Bus Selector1/3 -> Add2/2, Bus Creator2/3  "<R0_C2>"
  Bus Selector1/9 -> Bus Creator2/9  "<R0_TLC>"
  Average Filter (AvrgFlt)/1(Out) -> Bus Creator1/1  "L0_C0"
  Add/1 -> Switch/1
  [offset] -> Add/2
  Compare To Constant/1 -> Switch/2
  Bus Selector3/10 -> Bus Creator1/10  "<L0_LC>"
  Bus Selector3/8 -> Bus Creator1/8  "<L0_W>"
  Bus Selector3/7 -> Compare To Constant/1, Bus Creator1/7  "<L0_Type>"
  Bus Selector3/5 -> Bus Creator1/5  "<L0_VR>"
  Bus Selector3/6 -> Bus Creator1/6  "<L0_Q>"
  Bus Selector3/4 -> Bus Creator1/4  "<L0_C3>"
  Bus Selector3/3 -> Add2/1, Bus Creator1/3  "<L0_C2>"
  Bus Selector3/2 -> Bus Creator1/2  "<L0_C1>"
  Bus Selector3/1 -> Add/1, Switch/3  "<L0_C0>"
  bsL0Info/1 -> Bus Selector3/1, Road Width Calculation (RoadWCal)/1(RoadWCal_L0Info)
  Bus Creator1/1 -> bsL0Infoout/1  "bsL0Info"
  Bus Selector3/9 -> Bus Creator1/9  "<L0_TLC>"

== system D53_LKAS_JLU_20200910_1510/LL/LLOn/LDW/Heading Angle Detection (HdAgDet)/If Action Subsystem ==
  In1 : Inport
  Action Port : ActionPort  InitializeStates=reset  ActionType=then
  Gain : Gain  Gain=-1  OutDataTypeStr=single
  rad to deg : Gain  Gain=180/pi  OutDataTypeStr=single
  Out1 : Outport  InitialOutput=0
  wires:
  rad to deg/1 -> Out1/1
  Gain/1 -> rad to deg/1
  In1/1 -> Gain/1

== system D53_LKAS_JLU_20200910_1510/LL/LLOn/LDW/Heading Angle Detection (HdAgDet)/If Action Subsystem1 ==
  In1 : Inport
  Action Port : ActionPort  InitializeStates=reset  ActionType=elseif
  rad to deg : Gain  Gain=180/pi  OutDataTypeStr=single
  Out1 : Outport  InitialOutput=0
  wires:
  rad to deg/1 -> Out1/1
  In1/1 -> rad to deg/1

== system D53_LKAS_JLU_20200910_1510/LL/LLOn/LDW/Heading Angle Detection (HdAgDet)/If Action Subsystem2 ==
  Action Port : ActionPort  InitializeStates=reset  ActionType=else
  Constant : Constant  Value=0  OutDataTypeStr=single
  Out1 : Outport  InitialOutput=0
  wires:
  Constant/1 -> Out1/1

== system D53_LKAS_JLU_20200910_1510/LL/LLOn/LDW/Heading Angle Detection (HdAgDet)/Sum Condition ==
  In : Inport
  Sum : Inport  Port=2
  state = reset : EnablePort  StatesWhenEnabling=reset
  Add1 : Sum  OutDataTypeStr=single
  Data Type Conversion : DataTypeConversion  OutDataTypeStr=uint8
  Memory : Memory  InheritSampleTime=on
  Relational Operator : RelationalOperator  OutDataTypeStr=boolean  RndMeth=Nearest
  Saturation : Saturate  UpperLimit=600  LowerLimit=0
  Out : Outport  OutputWhenDisabled=reset  InitialOutput=0
  wires:
  Saturation/1 -> Relational Operator/1, Memory/1
  Data Type Conversion/1 -> Out/1
  Sum/1 -> Relational Operator/2
  In/1 -> Add1/1
  Add1/1 -> Saturation/1
  Memory/1 -> Add1/2
  Relational Operator/1 -> Data Type Conversion/1

== system D53_LKAS_JLU_20200910_1510/LL/LLOn/LKA/Driver Torque Addition (DTA)/Subsystem ==
  DTA_bsInInfoSyn : Inport
  DTA_bsLFClb : Inport  Port=2
  LKA_SampleTime : Inport  Port=3
  Enable : EnablePort
  Add : Sum
  Bus Selector2 : BusSelector  OutputSignals=bsVehMovInfo.ESC_VehSpd,bsEPSInfo.EPS_SW_Trq,bsLaneInfo.bsL0Info.L0_C0,bsLaneInfo.bsR0Info.R0_C0
  Bus Selector4 : BusSelector  OutputSignals=LL_LKASWAClb.LL_LKASWASyn_SWAaddMax,LL_LKASWAClb.LL_LKASWASyn_TrqMax,LL_LKASWAClb.LL_LKASWASyn_TrqSwaAddSwt,LL_LKASWAClb.LL_LKASWASyn_tiTrqSwaTime,LL_LKASWAClb.LL_LKASWASyn_tiTrqSwaRtTime,LL_LKASWAClb.LL_LKASWASyn_TrqSwaRateDiff
  Constant1 : Constant  Value=5  OutDataTypeStr=single
  Constant2 : Constant  Value=-5  OutDataTypeStr=single
  Divide1 : Product  Inputs=***
  Divide3 : Product  Inputs=**
  DriverSwaTrqAdd : MATLAB Function  TreatAsAtomicUnit=on
  LowPass : Subsystem
  LowPass1 : Subsystem
  Rate Limiter Dynamic : simulink/Discontinuities/Rate Limiter Dynamic
      settings: SourceProductName=Simulink
  Saturation : Saturate  UpperLimit=30  LowerLimit=-30
  Out1 : Outport  OutputWhenDisabled=reset  InitialOutput=0
  wires:
  DTA_bsLFClb/1 -> Bus Selector4/1
  Bus Selector4/2 -> DriverSwaTrqAdd/6(trqmax)  "<LL_LKASWASyn_TrqMax>"
  LKA_SampleTime/1 -> LowPass1/3(dT), LowPass/3(dT)
  Bus Selector2/3 -> DriverSwaTrqAdd/3(l0c0)  "<L0_C0>"
  Bus Selector4/5 -> LowPass1/1(T)  "<LL_LKASWASyn_tiTrqSwaRtTime>"
  Bus Selector2/1 -> DriverSwaTrqAdd/1(spd)  "<ESC_VehSpd>"
  Bus Selector4/6 -> Divide1/3  "<LL_LKASWASyn_TrqSwaRateDiff>"
  Bus Selector2/4 -> DriverSwaTrqAdd/4(r0c0)  "<R0_C0>"
  Bus Selector2/2 -> DriverSwaTrqAdd/2(trq)  "<EPS_SW_Trq>"
  Divide1/1 -> Add/2  "SWARateAdd"
  LowPass/1(y) -> LowPass1/2(u), Divide3/2  "TrqSWAAdd"
  Bus Selector4/4 -> LowPass/1(T)  "<LL_LKASWASyn_tiTrqSwaTime>"
  DTA_bsInInfoSyn/1 -> Bus Selector2/1
  Saturation/1 -> Divide1/2
  Rate Limiter Dynamic/1 -> Out1/1
  DriverSwaTrqAdd/1(Swaadd) -> LowPass/2(u)  "TrqSWAAddRaw"
  Constant1/1 -> Rate Limiter Dynamic/1
  Bus Selector4/1 -> DriverSwaTrqAdd/5(swaaddmax)  "<LL_LKASWASyn_SWAaddMax>"
  Constant2/1 -> Rate Limiter Dynamic/3
  Divide3/1 -> Add/1  "TrqSWAAdd"
  LowPass1/1(y) -> Saturation/1  "SWARateAdd"
  Bus Selector4/3 -> Divide1/1, Divide3/1  "<LL_LKASWASyn_TrqSwaAddSwt>"
  Add/1 -> Rate Limiter Dynamic/2

== system D53_LKAS_JLU_20200910_1510/LL/LLOn/LKA/Driver Torque Addition (DTA)/Subsystem1 ==
  DTA_bsInInfoSyn : Inport
  DTA_bsLFClb : Inport  Port=2
  Add1 : Sum  Inputs=-+
  Bus Selector : BusSelector  OutputSignals=bsEPSInfo.EPS_SW_Trq
  Bus Selector1 : BusSelector  OutputSignals=LL_LKASWAClb.LL_LKASWASyn_M3K,LL_LKASWAClb.LL_LKASWASyn_M0,LL_LKASWAClb.LL_LKASWASyn_M1,LL_LKASWAClb.LL_LKASWASyn_M2,LL_LKASWAClb.LL_LKASWASyn_T2
  Divide : Product  Inputs=**
  MATLAB Function : MATLAB Function  TreatAsAtomicUnit=on
  Moving Standard Deviation2 : Subsystem  TreatAsAtomicUnit=on
      mask Display: disp(['Moving' char(10) 'Standard' char(10) 'Deviation']);
  Saturation1 : Saturate  UpperLimit=0.2  LowerLimit=0
  Saturation2 : Saturate  UpperLimit=1  LowerLimit=0
  TickTime (TTime) : Subsystem
      mask Display:
      | port_label('output', 1, 'TTime');
      | color('blue');
      | text(0.98,0.9,'VCDC Block','horizontalAlignment','right');
      | color('black');
      | text(0.5,0.55,'Tick Time','horizontalAlignment','center');
      | text(0.5,0.4,'(TTime)','horizontalAlignment','center');
  Out1 : Outport
  wires:
  Saturation2/1 -> Out1/1
  DTA_bsLFClb/1 -> Bus Selector1/1
  DTA_bsInInfoSyn/1 -> Bus Selector/1
  Moving Standard Deviation2/1(Out1) -> Divide/1
  Bus Selector/1 -> Moving Standard Deviation2/1(In1)  "<EPS_SW_Trq>"
  Bus Selector1/4 -> MATLAB Function/3(M2)  "<LL_LKASWASyn_M2>"
  Bus Selector1/1 -> Divide/2  "<LL_LKASWASyn_M3K>"
  Add1/1 -> Saturation2/1
  Divide/1 -> Saturation1/1
  TickTime (TTime)/1(Out1) -> [T]
  Bus Selector1/5 -> MATLAB Function/5(T2)  "<LL_LKASWASyn_T2>"
  MATLAB Function/1(M) -> Add1/2
  Saturation1/1 -> Add1/1  "M3"
  [T] -> MATLAB Function/6(T)
  [PT1] -> MATLAB Function/4(T1)
  Bus Selector1/3 -> MATLAB Function/2(M1)  "<LL_LKASWASyn_M1>"
  Bus Selector1/2 -> MATLAB Function/1(M0)  "<LL_LKASWASyn_M0>"

== system D53_LKAS_JLU_20200910_1510/LL/LLOn/LKA/LKA Exit Processing (LKAExPrcs)/Exit Time 1 ==
  bsLKAInPInfo : Inport
  bsLKAClb : Inport  Port=2
  Abs : Abs
  Add : Sum
  Add2 : Sum  OutDataTypeStr=single
  Bus Selector1 : BusSelector  OutputSignals=LL_LKAExPrcs.LL_LKAExPrcs_tiExitTime1
  Bus Selector2 : BusSelector  OutputSignals=Pr_bsPrInfo.bsPrCrvtInfo.crPrvwCrvt
  Constant : Constant  Value=0.004  OutDataTypeStr=single
  Constant1 : Constant  Value=0.5  OutDataTypeStr=single
  Divide : Product  Inputs=***/
  Memory : Memory  InheritSampleTime=on
  Relational Operator4 : RelationalOperator  OutDataTypeStr=boolean  RndMeth=Nearest
  Saturation : Saturate  UpperLimit=0.004  LowerLimit=0
  Saturation2 : Saturate  UpperLimit=10  LowerLimit=0
  Exit1 : Outport
  wires:
  Bus Selector1/1 -> Divide/1, Add/1  "<LL_LKAExPrcs_tiExitTime1>"
  Saturation/1 -> Divide/3
  Add/1 -> Relational Operator4/2
  Abs/1 -> Saturation/1
  Divide/1 -> Add/2
  Bus Selector2/1 -> Abs/1  "<crPrvwCrvt>"
  Constant1/1 -> Divide/2
  Constant/1 -> Divide/4
  bsLKAInPInfo/1 -> Bus Selector2/1
  Relational Operator4/1 -> Exit1/1
  Memory/1 -> Add2/2
  Saturation2/1 -> Memory/1
  bsLKAClb/1 -> Bus Selector1/1
  Add2/1 -> Relational Operator4/1, Saturation2/1
  [LKA_SampleTime] -> Add2/1

== system D53_LKAS_JLU_20200910_1510/LL/LLOn/LKA/LKA Exit Processing (LKAExPrcs)/Exit Time 2 ==
  bsInInfoSyn : Inport
  bsLKAClb : Inport  Port=2
  bsLKAInPInfo : Inport  Port=3
  T1 : Inport  Port=4
  Abs : Abs
  Abs2 : Abs
  Abs3 : Abs
  Add : Sum
  Add1 : Sum
  Add2 : Sum  OutDataTypeStr=single
  Bus Selector : BusSelector  OutputSignals=LKA_Veh2CamW_C
  Bus Selector1 : BusSelector  OutputSignals=Pr_bsPrInfo.bsPrCrvtInfo.crPrvwCrvt
  Bus Selector2 : BusSelector  OutputSignals=bsLaneInfo.bsL0Info.L0_C0,bsLaneInfo.bsR0Info.R0_C0
  Bus Selector3 : BusSelector  OutputSignals=LL_LKAExPrcs.LL_LKAExPrcs_tiExitTime2
  Constant : Constant  Value=0.004  OutDataTypeStr=single
  Constant1 : Constant  Value=0.5  OutDataTypeStr=single
  Constant3 : Constant  Value=0.3  OutDataTypeStr=single
  Divide : Product  Inputs=***/
  Logical Operator1 : Logic  Inputs=3  AllPortsSameDT=off  OutDataTypeStr=boolean
  Memory : Memory  InheritSampleTime=on
  Relational Operator2 : RelationalOperator  OutDataTypeStr=boolean  RndMeth=Nearest
  Relational Operator3 : RelationalOperator  OutDataTypeStr=boolean  RndMeth=Nearest
  Relational Operator4 : RelationalOperator  OutDataTypeStr=boolean  RndMeth=Nearest
  Saturation : Saturate  UpperLimit=0.004  LowerLimit=0
  Saturation2 : Saturate  UpperLimit=10  LowerLimit=0
  Sum Condition1 : Subsystem
  Exit2 : Outport
  wires:
  bsLKAClb/1 -> Bus Selector3/1
  [LKA_ConstantClb] -> Bus Selector/1
  Bus Selector/1 -> Add/2  "<LKA_Veh2CamW_C>"
  Saturation/1 -> Divide/3
  Bus Selector3/1 -> Add1/1, Divide/1  "<LL_LKAExPrcs_tiExitTime2>"
  Divide/1 -> Add1/2
  Constant1/1 -> Divide/2
  Abs/1 -> Saturation/1
  Constant/1 -> Divide/4
  Add1/1 -> Sum Condition1/2(Time Exit 2)
  Bus Selector1/1 -> Abs/1  "<crPrvwCrvt>"
  bsLKAInPInfo/1 -> Bus Selector1/1
  bsInInfoSyn/1 -> Bus Selector2/1
  [LKA_SampleTime] -> Sum Condition1/1(Sample Time)
  Sum Condition1/1(Out) -> Exit2/1
  T1/1 -> Relational Operator4/2
  [LKA_SampleTime] -> Add2/1
  Memory/1 -> Add2/2
  Add2/1 -> Relational Operator4/1, Saturation2/1
  Relational Operator4/1 -> Logical Operator1/1
  Saturation2/1 -> Memory/1
  Constant3/1 -> Add/1
  Logical Operator1/1 -> Sum Condition1/Enable
  Relational Operator3/1 -> Logical Operator1/3
  Abs2/1 -> Relational Operator2/1
  Bus Selector2/1 -> Abs2/1  "<L0_C0>"
  Relational Operator2/1 -> Logical Operator1/2
  Abs3/1 -> Relational Operator3/1
  Bus Selector2/2 -> Abs3/1  "<R0_C0>"
  Add/1 -> Relational Operator2/2, Relational Operator3/2

== system D53_LKAS_JLU_20200910_1510/LL/LLOn/LKA/LKA Exit Processing (LKAExPrcs)/Exit Time 3 ==
  bsInInfoSyn : Inport
  bsLKAInPInfo : Inport  Port=2
  bsLKAClb : Inport  Port=3
  T1 : Inport  Port=4
  Abs2 : Abs
  Abs3 : Abs
  Abs4 : Abs
  Add : Sum
  Add2 : Sum  OutDataTypeStr=single
  Add4 : Sum
  Add5 : Sum  Inputs=+-
  Add6 : Sum
  Bus Selector : BusSelector  OutputSignals=LKA_Veh2CamW_C
  Bus Selector1 : BusSelector  OutputSignals=bsLaneInfo.bsL0Info.L0_C0,bsLaneInfo.bsR0Info.R0_C0
  Bus Selector2 : BusSelector  OutputSignals=bsLaneInfo.bsL0Info.L0_C0,bsLaneInfo.bsR0Info.R0_C0
  Bus Selector3 : BusSelector  OutputSignals=LL_LKAExPrcs.LL_LKAExPrcs_tiExitTime3,LL_LKAExPrcs.LL_LKAExPrcs_ExitC0Dvt,LL_LKAExPrcs.LL_LKAExPrcs_ExitC0Swt
  Bus Selector4 : BusSelector  OutputSignals=Pr_bsPrInfo.bsPrCrvtInfo.crPrvwCrvt
  Constant : Constant  Value=0.004  OutDataTypeStr=single
  Constant4 : Constant  Value=0.3  OutDataTypeStr=single
  Constant7 : Constant  Value=2  OutDataTypeStr=single
  Divide1 : Product  Inputs=**/
  Divide2 : Product  Inputs=*/
  Gain : Gain  Gain=0.25
  Logical Operator1 : Logic  Inputs=3  AllPortsSameDT=off  OutDataTypeStr=boolean
  Logical Operator2 : Logic  Inputs=4  AllPortsSameDT=off  OutDataTypeStr=boolean
  Memory : Memory  InheritSampleTime=on
  Moving Standard Deviation1 : Subsystem  TreatAsAtomicUnit=on
      mask Display: disp(['Moving' char(10) 'Standard' char(10) 'Deviation']);
  Moving Standard Deviation2 : Subsystem  TreatAsAtomicUnit=on
      mask Display: disp(['Moving' char(10) 'Standard' char(10) 'Deviation']);
  Relational Operator2 : RelationalOperator  OutDataTypeStr=boolean  RndMeth=Nearest
  Relational Operator3 : RelationalOperator  OutDataTypeStr=boolean  RndMeth=Nearest
  Relational Operator4 : RelationalOperator  OutDataTypeStr=boolean  RndMeth=Nearest
  Relational Operator5 : RelationalOperator  Operator=<=  OutDataTypeStr=boolean  RndMeth=Nearest
  Relational Operator6 : RelationalOperator  Operator=<=  OutDataTypeStr=boolean  RndMeth=Nearest
  Saturation : Saturate  UpperLimit=0.004  LowerLimit=0
  Saturation1 : Saturate  UpperLimit=5.5  LowerLimit=2.4
  Saturation2 : Saturate  UpperLimit=10  LowerLimit=0
  Sum Condition : Subsystem
  Sum Condition1 : Subsystem
  Exit3 : Outport
  wires:
  Add6/1 -> Divide2/1
  [LKA_SampleTime] -> Divide2/2
  Constant7/1 -> Divide1/1
  Bus Selector4/1 -> Abs4/1  "<crPrvwCrvt>"
  Saturation/1 -> Divide1/2
  Abs4/1 -> Saturation/1
  Divide1/1 -> Add6/2
  Constant/1 -> Divide1/3
  bsLKAInPInfo/1 -> Bus Selector4/1
  Moving Standard Deviation1/1(Out1) -> Relational Operator6/1
  Divide2/1 -> Sum Condition1/2(In1), Sum Condition/2(In1)
  Relational Operator6/1 -> Sum Condition1/1(In), Sum Condition1/Enable
  Sum Condition1/1(Out) -> Logical Operator2/2
  Sum Condition/1(Out) -> Logical Operator2/3
  Relational Operator5/1 -> Sum Condition/1(In), Sum Condition/Enable
  Gain/1 -> Add5/1
  Constant4/1 -> Add5/2
  Saturation1/1 -> Gain/1
  Add4/1 -> Saturation1/1
  Moving Standard Deviation2/1(Out1) -> Relational Operator5/1
  [LKA_ConstantClb] -> Bus Selector/1
  Bus Selector/1 -> Add/2  "<LKA_Veh2CamW_C>"
  Logical Operator2/1 -> Exit3/1
  Bus Selector1/1 -> Moving Standard Deviation2/1(In1)  "<L0_C0>"
  Bus Selector1/2 -> Moving Standard Deviation1/1(In1)  "<R0_C0>"
  bsLKAClb/1 -> Bus Selector3/1
  Bus Selector3/2 -> Relational Operator6/2, Relational Operator5/2  "<LL_LKAExPrcs_ExitC0Dvt>"
  bsInInfoSyn/1 -> Bus Selector1/1, Bus Selector2/1
  Bus Selector3/3 -> Logical Operator2/4  "<LL_LKAExPrcs_ExitC0Swt>"
  Bus Selector3/1 -> Add6/1  "<LL_LKAExPrcs_tiExitTime3>"
  Add/1 -> Relational Operator3/2, Relational Operator2/2
  Bus Selector2/2 -> Abs3/1  "<R0_C0>"
  Abs3/1 -> Relational Operator3/1, Add4/2
  Relational Operator2/1 -> Logical Operator1/2
  Bus Selector2/1 -> Abs2/1  "<L0_C0>"
  Abs2/1 -> Add4/1, Relational Operator2/1
  Relational Operator3/1 -> Logical Operator1/3
  Logical Operator1/1 -> Logical Operator2/1
  Add5/1 -> Add/1
  Saturation2/1 -> Memory/1
  Relational Operator4/1 -> Logical Operator1/1
  Add2/1 -> Saturation2/1, Relational Operator4/1
  Memory/1 -> Add2/2
  [LKA_SampleTime] -> Add2/1
  T1/1 -> Relational Operator4/2
